simulink model "LoFT_Example3"  (R2024b)
settings: Solver=ode4  StartTime=0.0  StopTime=300  FixedStep=simu.dt  RelTol=1e-3
undefined symbols (not defined in the file): body, circtime, Communication, D1, Delta, irkb, line, LoFT, p0, Pn, s, simu, trip_time, Turbwind, waves, wind
libraries: simulink x350, spsThreePhaseVIMeasurementLib x41, spsThreePhasePISectionLineLib x34, spsThreePhaseParallelRLCLoadLib x21, spsThreePhaseTransformerTwoWindingsLib x14, spsLoadFlowBusLib x10, spsThreePhaseDynamicLoadLib x9, spsSynchronousMachinepuStandardLib x7, spsExcitationSystemLib x7, spsSteamTurbineandGovernorLib x7, spsGenericPowerSystemStabilizerLib x7, spsMultiBandPowerSystemStabilizerLib x7
(part 46 of 49)

== system LoFT_Example3/FOWT System/Subsystem13/FOWT2/Aerodynamics and Local Control Systems/Local Control Systems/Subsystem1/Gain Scheduling ==
  In1 : Inport
  In3 : Inport  Port=2
  In2 : Inport  Port=3
  1-D Lookup Table1 : Lookup_n-D  NumberOfTableDimensions=1  BreakpointsForDimension1=Controller.R.PC_GS_angles  Table=Controller.R.PC_GS_KI  InternalRulePriority=Speed  RndMeth=Simplest
  1-D Lookup Table2 : Lookup_n-D  NumberOfTableDimensions=1  BreakpointsForDimension1=Controller.R.PC_GS_angles  Table=Controller.R.PC_GS_KP  InternalRulePriority=Speed  RndMeth=Simplest
  Add : Sum
  Add1 : Sum
  Constant1 : Constant  Value=90*pi/180
  Delay : Delay  DelayLength=1  InitialCondition=0
  Gain : Gain  Gain=simu.dt
  Product : Product
  Product1 : Product
  Saturation Dynamic : simulink/Discontinuities/Saturation Dynamic  OutMin=[]  OutMax=[]  OutDataTypeStr=Inherit: Same as second input  OutDataType=fixdt(1, 16)  OutScaling=2^-10  DoSatur=off
  Saturation1 : Saturate  UpperLimit=Controller.R.PC_GS_KI(end)  LowerLimit=Controller.R.PC_GS_KI(1)
  Saturation3 : Saturate  UpperLimit=Controller.R.PC_GS_KP(end)  LowerLimit=Controller.R.PC_GS_KP(1)
  Out1 : Outport
  wires:
  Product/1 -> Add1/1
  Add1/1 -> Out1/1
  Delay/1 -> Add/2
  Saturation Dynamic/1 -> Delay/1, Add1/2
  Constant1/1 -> Saturation Dynamic/1
  In3/1 -> Saturation Dynamic/3
  Add/1 -> Saturation Dynamic/2
  Gain/1 -> Add/1
  Product1/1 -> Gain/1
  Saturation1/1 -> Product1/2
  Saturation3/1 -> Product/2
  In1/1 -> Product1/1, Product/1
  In2/1 -> 1-D Lookup Table2/1, 1-D Lookup Table1/1
  1-D Lookup Table2/1 -> Saturation3/1
  1-D Lookup Table1/1 -> Saturation1/1

== system LoFT_Example3/FOWT System/Subsystem13/FOWT3/Aerodynamics and Local Control Systems/Local Control Systems/Subsystem1/Gain Scheduling ==
  In1 : Inport
  In3 : Inport  Port=2
  In2 : Inport  Port=3
  1-D Lookup Table1 : Lookup_n-D  NumberOfTableDimensions=1  BreakpointsForDimension1=Controller.R.PC_GS_angles  Table=Controller.R.PC_GS_KI  InternalRulePriority=Speed  RndMeth=Simplest
  1-D Lookup Table2 : Lookup_n-D  NumberOfTableDimensions=1  BreakpointsForDimension1=Controller.R.PC_GS_angles  Table=Controller.R.PC_GS_KP  InternalRulePriority=Speed  RndMeth=Simplest
  Add : Sum
  Add1 : Sum
  Constant1 : Constant  Value=90*pi/180
  Delay : Delay  DelayLength=1  InitialCondition=0
  Gain : Gain  Gain=simu.dt
  Product : Product
  Product1 : Product
  Saturation Dynamic : simulink/Discontinuities/Saturation Dynamic  OutMin=[]  OutMax=[]  OutDataTypeStr=Inherit: Same as second input  OutDataType=fixdt(1, 16)  OutScaling=2^-10  DoSatur=off
  Saturation1 : Saturate  UpperLimit=Controller.R.PC_GS_KI(end)  LowerLimit=Controller.R.PC_GS_KI(1)
  Saturation3 : Saturate  UpperLimit=Controller.R.PC_GS_KP(end)  LowerLimit=Controller.R.PC_GS_KP(1)
  Out1 : Outport
  wires:
  1-D Lookup Table1/1 -> Saturation1/1
  1-D Lookup Table2/1 -> Saturation3/1
  In2/1 -> 1-D Lookup Table1/1, 1-D Lookup Table2/1
  In1/1 -> Product/1, Product1/1
  Saturation3/1 -> Product/2
  Saturation1/1 -> Product1/2
  Product1/1 -> Gain/1
  Gain/1 -> Add/1
  Add/1 -> Saturation Dynamic/2
  In3/1 -> Saturation Dynamic/3
  Constant1/1 -> Saturation Dynamic/1
  Saturation Dynamic/1 -> Add1/2, Delay/1
  Delay/1 -> Add/2
  Add1/1 -> Out1/1
  Product/1 -> Add1/1

== system LoFT_Example3/FOWT System/Subsystem13/FOWT4/Aerodynamics and Local Control Systems/Local Control Systems/Subsystem1/Gain Scheduling ==
  In1 : Inport
  In3 : Inport  Port=2
  In2 : Inport  Port=3
  1-D Lookup Table1 : Lookup_n-D  NumberOfTableDimensions=1  BreakpointsForDimension1=Controller.R.PC_GS_angles  Table=Controller.R.PC_GS_KI  InternalRulePriority=Speed  RndMeth=Simplest
  1-D Lookup Table2 : Lookup_n-D  NumberOfTableDimensions=1  BreakpointsForDimension1=Controller.R.PC_GS_angles  Table=Controller.R.PC_GS_KP  InternalRulePriority=Speed  RndMeth=Simplest
  Add : Sum
  Add1 : Sum
  Constant1 : Constant  Value=90*pi/180
  Delay : Delay  DelayLength=1  InitialCondition=0
  Gain : Gain  Gain=simu.dt
  Product : Product
  Product1 : Product
  Saturation Dynamic : simulink/Discontinuities/Saturation Dynamic  OutMin=[]  OutMax=[]  OutDataTypeStr=Inherit: Same as second input  OutDataType=fixdt(1, 16)  OutScaling=2^-10  DoSatur=off
  Saturation1 : Saturate  UpperLimit=Controller.R.PC_GS_KI(end)  LowerLimit=Controller.R.PC_GS_KI(1)
  Saturation3 : Saturate  UpperLimit=Controller.R.PC_GS_KP(end)  LowerLimit=Controller.R.PC_GS_KP(1)
  Out1 : Outport
  wires:
  Product/1 -> Add1/1
  Add1/1 -> Out1/1
  Delay/1 -> Add/2
  Saturation Dynamic/1 -> Delay/1, Add1/2
  Constant1/1 -> Saturation Dynamic/1
  In3/1 -> Saturation Dynamic/3
  Add/1 -> Saturation Dynamic/2
  Gain/1 -> Add/1
  Product1/1 -> Gain/1
  Saturation1/1 -> Product1/2
  Saturation3/1 -> Product/2
  In1/1 -> Product1/1, Product/1
  In2/1 -> 1-D Lookup Table2/1, 1-D Lookup Table1/1
  1-D Lookup Table2/1 -> Saturation3/1
  1-D Lookup Table1/1 -> Saturation1/1

== system LoFT_Example3/FOWT System/Subsystem13/FOWT5/Aerodynamics and Local Control Systems/Local Control Systems/Subsystem1/Gain Scheduling ==
  In1 : Inport
  In3 : Inport  Port=2
  In2 : Inport  Port=3
  1-D Lookup Table1 : Lookup_n-D  NumberOfTableDimensions=1  BreakpointsForDimension1=Controller.R.PC_GS_angles  Table=Controller.R.PC_GS_KI  InternalRulePriority=Speed  RndMeth=Simplest
  1-D Lookup Table2 : Lookup_n-D  NumberOfTableDimensions=1  BreakpointsForDimension1=Controller.R.PC_GS_angles  Table=Controller.R.PC_GS_KP  InternalRulePriority=Speed  RndMeth=Simplest
  Add : Sum
  Add1 : Sum
  Constant1 : Constant  Value=90*pi/180
  Delay : Delay  DelayLength=1  InitialCondition=0
  Gain : Gain  Gain=simu.dt
  Product : Product
  Product1 : Product
  Saturation Dynamic : simulink/Discontinuities/Saturation Dynamic  OutMin=[]  OutMax=[]  OutDataTypeStr=Inherit: Same as second input  OutDataType=fixdt(1, 16)  OutScaling=2^-10  DoSatur=off
  Saturation1 : Saturate  UpperLimit=Controller.R.PC_GS_KI(end)  LowerLimit=Controller.R.PC_GS_KI(1)
  Saturation3 : Saturate  UpperLimit=Controller.R.PC_GS_KP(end)  LowerLimit=Controller.R.PC_GS_KP(1)
  Out1 : Outport
  wires:
  1-D Lookup Table1/1 -> Saturation1/1
  1-D Lookup Table2/1 -> Saturation3/1
  In2/1 -> 1-D Lookup Table1/1, 1-D Lookup Table2/1
  In1/1 -> Product/1, Product1/1
  Saturation3/1 -> Product/2
  Saturation1/1 -> Product1/2
  Product1/1 -> Gain/1
  Gain/1 -> Add/1
  Add/1 -> Saturation Dynamic/2
  In3/1 -> Saturation Dynamic/3
  Constant1/1 -> Saturation Dynamic/1
  Saturation Dynamic/1 -> Add1/2, Delay/1
  Delay/1 -> Add/2
  Add1/1 -> Out1/1
  Product/1 -> Add1/1

== system LoFT_Example3/FOWT System/Subsystem13/FOWT6/Aerodynamics and Local Control Systems/Local Control Systems/Subsystem1/Gain Scheduling ==
  In1 : Inport
  In3 : Inport  Port=2
  In2 : Inport  Port=3
  1-D Lookup Table1 : Lookup_n-D  NumberOfTableDimensions=1  BreakpointsForDimension1=Controller.R.PC_GS_angles  Table=Controller.R.PC_GS_KI  InternalRulePriority=Speed  RndMeth=Simplest
  1-D Lookup Table2 : Lookup_n-D  NumberOfTableDimensions=1  BreakpointsForDimension1=Controller.R.PC_GS_angles  Table=Controller.R.PC_GS_KP  InternalRulePriority=Speed  RndMeth=Simplest
  Add : Sum
  Add1 : Sum
  Constant1 : Constant  Value=90*pi/180
  Delay : Delay  DelayLength=1  InitialCondition=0
  Gain : Gain  Gain=simu.dt
  Product : Product
  Product1 : Product
  Saturation Dynamic : simulink/Discontinuities/Saturation Dynamic  OutMin=[]  OutMax=[]  OutDataTypeStr=Inherit: Same as second input  OutDataType=fixdt(1, 16)  OutScaling=2^-10  DoSatur=off
  Saturation1 : Saturate  UpperLimit=Controller.R.PC_GS_KI(end)  LowerLimit=Controller.R.PC_GS_KI(1)
  Saturation3 : Saturate  UpperLimit=Controller.R.PC_GS_KP(end)  LowerLimit=Controller.R.PC_GS_KP(1)
  Out1 : Outport
  wires:
  Product/1 -> Add1/1
  Add1/1 -> Out1/1
  Delay/1 -> Add/2
  Saturation Dynamic/1 -> Delay/1, Add1/2
  Constant1/1 -> Saturation Dynamic/1
  In3/1 -> Saturation Dynamic/3
  Add/1 -> Saturation Dynamic/2
  Gain/1 -> Add/1
  Product1/1 -> Gain/1
  Saturation1/1 -> Product1/2
  Saturation3/1 -> Product/2
  In1/1 -> Product1/1, Product/1
  In2/1 -> 1-D Lookup Table2/1, 1-D Lookup Table1/1
  1-D Lookup Table2/1 -> Saturation3/1
  1-D Lookup Table1/1 -> Saturation1/1

== system LoFT_Example3/FOWT System/Subsystem13/FOWT7/Aerodynamics and Local Control Systems/Local Control Systems/Subsystem1/Gain Scheduling ==
  In1 : Inport
  In3 : Inport  Port=2
  In2 : Inport  Port=3
  1-D Lookup Table1 : Lookup_n-D  NumberOfTableDimensions=1  BreakpointsForDimension1=Controller.R.PC_GS_angles  Table=Controller.R.PC_GS_KI  InternalRulePriority=Speed  RndMeth=Simplest
  1-D Lookup Table2 : Lookup_n-D  NumberOfTableDimensions=1  BreakpointsForDimension1=Controller.R.PC_GS_angles  Table=Controller.R.PC_GS_KP  InternalRulePriority=Speed  RndMeth=Simplest
  Add : Sum
  Add1 : Sum
  Constant1 : Constant  Value=90*pi/180
  Delay : Delay  DelayLength=1  InitialCondition=0
  Gain : Gain  Gain=simu.dt
  Product : Product
  Product1 : Product
  Saturation Dynamic : simulink/Discontinuities/Saturation Dynamic  OutMin=[]  OutMax=[]  OutDataTypeStr=Inherit: Same as second input  OutDataType=fixdt(1, 16)  OutScaling=2^-10  DoSatur=off
  Saturation1 : Saturate  UpperLimit=Controller.R.PC_GS_KI(end)  LowerLimit=Controller.R.PC_GS_KI(1)
  Saturation3 : Saturate  UpperLimit=Controller.R.PC_GS_KP(end)  LowerLimit=Controller.R.PC_GS_KP(1)
  Out1 : Outport
  wires:
  1-D Lookup Table1/1 -> Saturation1/1
  1-D Lookup Table2/1 -> Saturation3/1
  In2/1 -> 1-D Lookup Table1/1, 1-D Lookup Table2/1
  In1/1 -> Product/1, Product1/1
  Saturation3/1 -> Product/2
  Saturation1/1 -> Product1/2
  Product1/1 -> Gain/1
  Gain/1 -> Add/1
  Add/1 -> Saturation Dynamic/2
  In3/1 -> Saturation Dynamic/3
  Constant1/1 -> Saturation Dynamic/1
  Saturation Dynamic/1 -> Add1/2, Delay/1
  Delay/1 -> Add/2
  Add1/1 -> Out1/1
  Product/1 -> Add1/1

== system LoFT_Example3/FOWT System/Subsystem13/FOWT8/Aerodynamics and Local Control Systems/Local Control Systems/Subsystem1/Gain Scheduling ==
  In1 : Inport
  In3 : Inport  Port=2
  In2 : Inport  Port=3
  1-D Lookup Table1 : Lookup_n-D  NumberOfTableDimensions=1  BreakpointsForDimension1=Controller.R.PC_GS_angles  Table=Controller.R.PC_GS_KI  InternalRulePriority=Speed  RndMeth=Simplest
  1-D Lookup Table2 : Lookup_n-D  NumberOfTableDimensions=1  BreakpointsForDimension1=Controller.R.PC_GS_angles  Table=Controller.R.PC_GS_KP  InternalRulePriority=Speed  RndMeth=Simplest
  Add : Sum
  Add1 : Sum
  Constant1 : Constant  Value=90*pi/180
  Delay : Delay  DelayLength=1  InitialCondition=0
  Gain : Gain  Gain=simu.dt
  Product : Product
  Product1 : Product
  Saturation Dynamic : simulink/Discontinuities/Saturation Dynamic  OutMin=[]  OutMax=[]  OutDataTypeStr=Inherit: Same as second input  OutDataType=fixdt(1, 16)  OutScaling=2^-10  DoSatur=off
  Saturation1 : Saturate  UpperLimit=Controller.R.PC_GS_KI(end)  LowerLimit=Controller.R.PC_GS_KI(1)
  Saturation3 : Saturate  UpperLimit=Controller.R.PC_GS_KP(end)  LowerLimit=Controller.R.PC_GS_KP(1)
  Out1 : Outport
  wires:
  Product/1 -> Add1/1
  Add1/1 -> Out1/1
  Delay/1 -> Add/2
  Saturation Dynamic/1 -> Delay/1, Add1/2
  Constant1/1 -> Saturation Dynamic/1
  In3/1 -> Saturation Dynamic/3
  Add/1 -> Saturation Dynamic/2
  Gain/1 -> Add/1
  Product1/1 -> Gain/1
  Saturation1/1 -> Product1/2
  Saturation3/1 -> Product/2
  In1/1 -> Product1/1, Product/1
  In2/1 -> 1-D Lookup Table2/1, 1-D Lookup Table1/1
  1-D Lookup Table2/1 -> Saturation3/1
  1-D Lookup Table1/1 -> Saturation1/1

== system LoFT_Example3/FOWT System/Subsystem13/FOWT9/Aerodynamics and Local Control Systems/Local Control Systems/Subsystem1/Gain Scheduling ==
  In1 : Inport
  In3 : Inport  Port=2
  In2 : Inport  Port=3
  1-D Lookup Table1 : Lookup_n-D  NumberOfTableDimensions=1  BreakpointsForDimension1=Controller.R.PC_GS_angles  Table=Controller.R.PC_GS_KI  InternalRulePriority=Speed  RndMeth=Simplest
  1-D Lookup Table2 : Lookup_n-D  NumberOfTableDimensions=1  BreakpointsForDimension1=Controller.R.PC_GS_angles  Table=Controller.R.PC_GS_KP  InternalRulePriority=Speed  RndMeth=Simplest
  Add : Sum
  Add1 : Sum
  Constant1 : Constant  Value=90*pi/180
  Delay : Delay  DelayLength=1  InitialCondition=0
  Gain : Gain  Gain=simu.dt
  Product : Product
  Product1 : Product
  Saturation Dynamic : simulink/Discontinuities/Saturation Dynamic  OutMin=[]  OutMax=[]  OutDataTypeStr=Inherit: Same as second input  OutDataType=fixdt(1, 16)  OutScaling=2^-10  DoSatur=off
  Saturation1 : Saturate  UpperLimit=Controller.R.PC_GS_KI(end)  LowerLimit=Controller.R.PC_GS_KI(1)
  Saturation3 : Saturate  UpperLimit=Controller.R.PC_GS_KP(end)  LowerLimit=Controller.R.PC_GS_KP(1)
  Out1 : Outport
  wires:
  1-D Lookup Table1/1 -> Saturation1/1
  1-D Lookup Table2/1 -> Saturation3/1
  In2/1 -> 1-D Lookup Table1/1, 1-D Lookup Table2/1
  In1/1 -> Product/1, Product1/1
  Saturation3/1 -> Product/2
  Saturation1/1 -> Product1/2
  Product1/1 -> Gain/1
  Gain/1 -> Add/1
  Add/1 -> Saturation Dynamic/2
  In3/1 -> Saturation Dynamic/3
  Constant1/1 -> Saturation Dynamic/1
  Saturation Dynamic/1 -> Add1/2, Delay/1
  Delay/1 -> Add/2
  Add1/1 -> Out1/1
  Product/1 -> Add1/1

== system LoFT_Example3/FOWT System/Subsystem2/FOWT1/Aerodynamics and Local Control Systems/Local Control Systems/Subsystem1/Gain Scheduling ==
  In1 : Inport
  In3 : Inport  Port=2
  In2 : Inport  Port=3
  1-D Lookup Table1 : Lookup_n-D  NumberOfTableDimensions=1  BreakpointsForDimension1=Controller.R.PC_GS_angles  Table=Controller.R.PC_GS_KI  InternalRulePriority=Speed  RndMeth=Simplest
  1-D Lookup Table2 : Lookup_n-D  NumberOfTableDimensions=1  BreakpointsForDimension1=Controller.R.PC_GS_angles  Table=Controller.R.PC_GS_KP  InternalRulePriority=Speed  RndMeth=Simplest
  Add : Sum
  Add1 : Sum
  Constant1 : Constant  Value=90*pi/180
  Delay : Delay  DelayLength=1  InitialCondition=0
  Gain : Gain  Gain=simu.dt
  Product : Product
  Product1 : Product
  Saturation Dynamic : simulink/Discontinuities/Saturation Dynamic  OutMin=[]  OutMax=[]  OutDataTypeStr=Inherit: Same as second input  OutDataType=fixdt(1, 16)  OutScaling=2^-10  DoSatur=off
  Saturation1 : Saturate  UpperLimit=Controller.R.PC_GS_KI(end)  LowerLimit=Controller.R.PC_GS_KI(1)
  Saturation3 : Saturate  UpperLimit=Controller.R.PC_GS_KP(end)  LowerLimit=Controller.R.PC_GS_KP(1)
  Out1 : Outport
  wires:
  1-D Lookup Table1/1 -> Saturation1/1
  1-D Lookup Table2/1 -> Saturation3/1
  In2/1 -> 1-D Lookup Table1/1, 1-D Lookup Table2/1
  In1/1 -> Product/1, Product1/1
  Saturation3/1 -> Product/2
  Saturation1/1 -> Product1/2
  Product1/1 -> Gain/1
  Gain/1 -> Add/1
  Add/1 -> Saturation Dynamic/2
  In3/1 -> Saturation Dynamic/3
  Constant1/1 -> Saturation Dynamic/1
  Saturation Dynamic/1 -> Add1/2, Delay/1
  Delay/1 -> Add/2
  Add1/1 -> Out1/1
  Product/1 -> Add1/1

== system LoFT_Example3/FOWT System/Subsystem2/FOWT10/Aerodynamics and Local Control Systems/Local Control Systems/Subsystem1/Gain Scheduling ==
  In1 : Inport
  In3 : Inport  Port=2
  In2 : Inport  Port=3
  1-D Lookup Table1 : Lookup_n-D  NumberOfTableDimensions=1  BreakpointsForDimension1=Controller.R.PC_GS_angles  Table=Controller.R.PC_GS_KI  InternalRulePriority=Speed  RndMeth=Simplest
  1-D Lookup Table2 : Lookup_n-D  NumberOfTableDimensions=1  BreakpointsForDimension1=Controller.R.PC_GS_angles  Table=Controller.R.PC_GS_KP  InternalRulePriority=Speed  RndMeth=Simplest
  Add : Sum
  Add1 : Sum
  Constant1 : Constant  Value=90*pi/180
  Delay : Delay  DelayLength=1  InitialCondition=0
  Gain : Gain  Gain=simu.dt
  Product : Product
  Product1 : Product
  Saturation Dynamic : simulink/Discontinuities/Saturation Dynamic  OutMin=[]  OutMax=[]  OutDataTypeStr=Inherit: Same as second input  OutDataType=fixdt(1, 16)  OutScaling=2^-10  DoSatur=off
  Saturation1 : Saturate  UpperLimit=Controller.R.PC_GS_KI(end)  LowerLimit=Controller.R.PC_GS_KI(1)
  Saturation3 : Saturate  UpperLimit=Controller.R.PC_GS_KP(end)  LowerLimit=Controller.R.PC_GS_KP(1)
  Out1 : Outport
  wires:
  Product/1 -> Add1/1
  Add1/1 -> Out1/1
  Delay/1 -> Add/2
  Saturation Dynamic/1 -> Delay/1, Add1/2
  Constant1/1 -> Saturation Dynamic/1
  In3/1 -> Saturation Dynamic/3
  Add/1 -> Saturation Dynamic/2
  Gain/1 -> Add/1
  Product1/1 -> Gain/1
  Saturation1/1 -> Product1/2
  Saturation3/1 -> Product/2
  In1/1 -> Product1/1, Product/1
  In2/1 -> 1-D Lookup Table2/1, 1-D Lookup Table1/1
  1-D Lookup Table2/1 -> Saturation3/1
  1-D Lookup Table1/1 -> Saturation1/1

== system LoFT_Example3/FOWT System/Subsystem2/FOWT2/Aerodynamics and Local Control Systems/Local Control Systems/Subsystem1/Gain Scheduling ==
  In1 : Inport
  In3 : Inport  Port=2
  In2 : Inport  Port=3
  1-D Lookup Table1 : Lookup_n-D  NumberOfTableDimensions=1  BreakpointsForDimension1=Controller.R.PC_GS_angles  Table=Controller.R.PC_GS_KI  InternalRulePriority=Speed  RndMeth=Simplest
  1-D Lookup Table2 : Lookup_n-D  NumberOfTableDimensions=1  BreakpointsForDimension1=Controller.R.PC_GS_angles  Table=Controller.R.PC_GS_KP  InternalRulePriority=Speed  RndMeth=Simplest
  Add : Sum
  Add1 : Sum
  Constant1 : Constant  Value=90*pi/180
  Delay : Delay  DelayLength=1  InitialCondition=0
  Gain : Gain  Gain=simu.dt
  Product : Product
  Product1 : Product
  Saturation Dynamic : simulink/Discontinuities/Saturation Dynamic  OutMin=[]  OutMax=[]  OutDataTypeStr=Inherit: Same as second input  OutDataType=fixdt(1, 16)  OutScaling=2^-10  DoSatur=off
  Saturation1 : Saturate  UpperLimit=Controller.R.PC_GS_KI(end)  LowerLimit=Controller.R.PC_GS_KI(1)
  Saturation3 : Saturate  UpperLimit=Controller.R.PC_GS_KP(end)  LowerLimit=Controller.R.PC_GS_KP(1)
  Out1 : Outport
  wires:
  Product/1 -> Add1/1
  Add1/1 -> Out1/1
  Delay/1 -> Add/2
  Saturation Dynamic/1 -> Delay/1, Add1/2
  Constant1/1 -> Saturation Dynamic/1
  In3/1 -> Saturation Dynamic/3
  Add/1 -> Saturation Dynamic/2
  Gain/1 -> Add/1
  Product1/1 -> Gain/1
  Saturation1/1 -> Product1/2
  Saturation3/1 -> Product/2
  In1/1 -> Product1/1, Product/1
  In2/1 -> 1-D Lookup Table2/1, 1-D Lookup Table1/1
  1-D Lookup Table2/1 -> Saturation3/1
  1-D Lookup Table1/1 -> Saturation1/1

== system LoFT_Example3/FOWT System/Subsystem2/FOWT3/Aerodynamics and Local Control Systems/Local Control Systems/Subsystem1/Gain Scheduling ==
  In1 : Inport
  In3 : Inport  Port=2
  In2 : Inport  Port=3
  1-D Lookup Table1 : Lookup_n-D  NumberOfTableDimensions=1  BreakpointsForDimension1=Controller.R.PC_GS_angles  Table=Controller.R.PC_GS_KI  InternalRulePriority=Speed  RndMeth=Simplest
  1-D Lookup Table2 : Lookup_n-D  NumberOfTableDimensions=1  BreakpointsForDimension1=Controller.R.PC_GS_angles  Table=Controller.R.PC_GS_KP  InternalRulePriority=Speed  RndMeth=Simplest
  Add : Sum
  Add1 : Sum
  Constant1 : Constant  Value=90*pi/180
  Delay : Delay  DelayLength=1  InitialCondition=0
  Gain : Gain  Gain=simu.dt
  Product : Product
  Product1 : Product
  Saturation Dynamic : simulink/Discontinuities/Saturation Dynamic  OutMin=[]  OutMax=[]  OutDataTypeStr=Inherit: Same as second input  OutDataType=fixdt(1, 16)  OutScaling=2^-10  DoSatur=off
  Saturation1 : Saturate  UpperLimit=Controller.R.PC_GS_KI(end)  LowerLimit=Controller.R.PC_GS_KI(1)
  Saturation3 : Saturate  UpperLimit=Controller.R.PC_GS_KP(end)  LowerLimit=Controller.R.PC_GS_KP(1)
  Out1 : Outport
  wires:
  1-D Lookup Table1/1 -> Saturation1/1
  1-D Lookup Table2/1 -> Saturation3/1
  In2/1 -> 1-D Lookup Table1/1, 1-D Lookup Table2/1
  In1/1 -> Product/1, Product1/1
  Saturation3/1 -> Product/2
  Saturation1/1 -> Product1/2
  Product1/1 -> Gain/1
  Gain/1 -> Add/1
  Add/1 -> Saturation Dynamic/2
  In3/1 -> Saturation Dynamic/3
  Constant1/1 -> Saturation Dynamic/1
  Saturation Dynamic/1 -> Add1/2, Delay/1
  Delay/1 -> Add/2
  Add1/1 -> Out1/1
  Product/1 -> Add1/1

== system LoFT_Example3/FOWT System/Subsystem2/FOWT4/Aerodynamics and Local Control Systems/Local Control Systems/Subsystem1/Gain Scheduling ==
  In1 : Inport
  In3 : Inport  Port=2
  In2 : Inport  Port=3
  1-D Lookup Table1 : Lookup_n-D  NumberOfTableDimensions=1  BreakpointsForDimension1=Controller.R.PC_GS_angles  Table=Controller.R.PC_GS_KI  InternalRulePriority=Speed  RndMeth=Simplest
  1-D Lookup Table2 : Lookup_n-D  NumberOfTableDimensions=1  BreakpointsForDimension1=Controller.R.PC_GS_angles  Table=Controller.R.PC_GS_KP  InternalRulePriority=Speed  RndMeth=Simplest
  Add : Sum
  Add1 : Sum
  Constant1 : Constant  Value=90*pi/180
  Delay : Delay  DelayLength=1  InitialCondition=0
  Gain : Gain  Gain=simu.dt
  Product : Product
  Product1 : Product
  Saturation Dynamic : simulink/Discontinuities/Saturation Dynamic  OutMin=[]  OutMax=[]  OutDataTypeStr=Inherit: Same as second input  OutDataType=fixdt(1, 16)  OutScaling=2^-10  DoSatur=off
  Saturation1 : Saturate  UpperLimit=Controller.R.PC_GS_KI(end)  LowerLimit=Controller.R.PC_GS_KI(1)
  Saturation3 : Saturate  UpperLimit=Controller.R.PC_GS_KP(end)  LowerLimit=Controller.R.PC_GS_KP(1)
  Out1 : Outport
  wires:
  Product/1 -> Add1/1
  Add1/1 -> Out1/1
  Delay/1 -> Add/2
  Saturation Dynamic/1 -> Delay/1, Add1/2
  Constant1/1 -> Saturation Dynamic/1
  In3/1 -> Saturation Dynamic/3
  Add/1 -> Saturation Dynamic/2
  Gain/1 -> Add/1
  Product1/1 -> Gain/1
  Saturation1/1 -> Product1/2
  Saturation3/1 -> Product/2
  In1/1 -> Product1/1, Product/1
  In2/1 -> 1-D Lookup Table2/1, 1-D Lookup Table1/1
  1-D Lookup Table2/1 -> Saturation3/1
  1-D Lookup Table1/1 -> Saturation1/1

== system LoFT_Example3/FOWT System/Subsystem2/FOWT5/Aerodynamics and Local Control Systems/Local Control Systems/Subsystem1/Gain Scheduling ==
  In1 : Inport
  In3 : Inport  Port=2
  In2 : Inport  Port=3
  1-D Lookup Table1 : Lookup_n-D  NumberOfTableDimensions=1  BreakpointsForDimension1=Controller.R.PC_GS_angles  Table=Controller.R.PC_GS_KI  InternalRulePriority=Speed  RndMeth=Simplest
  1-D Lookup Table2 : Lookup_n-D  NumberOfTableDimensions=1  BreakpointsForDimension1=Controller.R.PC_GS_angles  Table=Controller.R.PC_GS_KP  InternalRulePriority=Speed  RndMeth=Simplest
  Add : Sum
  Add1 : Sum
  Constant1 : Constant  Value=90*pi/180
  Delay : Delay  DelayLength=1  InitialCondition=0
  Gain : Gain  Gain=simu.dt
  Product : Product
  Product1 : Product
  Saturation Dynamic : simulink/Discontinuities/Saturation Dynamic  OutMin=[]  OutMax=[]  OutDataTypeStr=Inherit: Same as second input  OutDataType=fixdt(1, 16)  OutScaling=2^-10  DoSatur=off
  Saturation1 : Saturate  UpperLimit=Controller.R.PC_GS_KI(end)  LowerLimit=Controller.R.PC_GS_KI(1)
  Saturation3 : Saturate  UpperLimit=Controller.R.PC_GS_KP(end)  LowerLimit=Controller.R.PC_GS_KP(1)
  Out1 : Outport
  wires:
  1-D Lookup Table1/1 -> Saturation1/1
  1-D Lookup Table2/1 -> Saturation3/1
  In2/1 -> 1-D Lookup Table1/1, 1-D Lookup Table2/1
  In1/1 -> Product/1, Product1/1
  Saturation3/1 -> Product/2
  Saturation1/1 -> Product1/2
  Product1/1 -> Gain/1
  Gain/1 -> Add/1
  Add/1 -> Saturation Dynamic/2
  In3/1 -> Saturation Dynamic/3
  Constant1/1 -> Saturation Dynamic/1
  Saturation Dynamic/1 -> Add1/2, Delay/1
  Delay/1 -> Add/2
  Add1/1 -> Out1/1
  Product/1 -> Add1/1

== system LoFT_Example3/FOWT System/Subsystem2/FOWT6/Aerodynamics and Local Control Systems/Local Control Systems/Subsystem1/Gain Scheduling ==
  In1 : Inport
  In3 : Inport  Port=2
  In2 : Inport  Port=3
  1-D Lookup Table1 : Lookup_n-D  NumberOfTableDimensions=1  BreakpointsForDimension1=Controller.R.PC_GS_angles  Table=Controller.R.PC_GS_KI  InternalRulePriority=Speed  RndMeth=Simplest
  1-D Lookup Table2 : Lookup_n-D  NumberOfTableDimensions=1  BreakpointsForDimension1=Controller.R.PC_GS_angles  Table=Controller.R.PC_GS_KP  InternalRulePriority=Speed  RndMeth=Simplest
  Add : Sum
  Add1 : Sum
  Constant1 : Constant  Value=90*pi/180
  Delay : Delay  DelayLength=1  InitialCondition=0
  Gain : Gain  Gain=simu.dt
  Product : Product
  Product1 : Product
  Saturation Dynamic : simulink/Discontinuities/Saturation Dynamic  OutMin=[]  OutMax=[]  OutDataTypeStr=Inherit: Same as second input  OutDataType=fixdt(1, 16)  OutScaling=2^-10  DoSatur=off
  Saturation1 : Saturate  UpperLimit=Controller.R.PC_GS_KI(end)  LowerLimit=Controller.R.PC_GS_KI(1)
  Saturation3 : Saturate  UpperLimit=Controller.R.PC_GS_KP(end)  LowerLimit=Controller.R.PC_GS_KP(1)
  Out1 : Outport
  wires:
  Product/1 -> Add1/1
  Add1/1 -> Out1/1
  Delay/1 -> Add/2
  Saturation Dynamic/1 -> Delay/1, Add1/2
  Constant1/1 -> Saturation Dynamic/1
  In3/1 -> Saturation Dynamic/3
  Add/1 -> Saturation Dynamic/2
  Gain/1 -> Add/1
  Product1/1 -> Gain/1
  Saturation1/1 -> Product1/2
  Saturation3/1 -> Product/2
  In1/1 -> Product1/1, Product/1
  In2/1 -> 1-D Lookup Table2/1, 1-D Lookup Table1/1
  1-D Lookup Table2/1 -> Saturation3/1
  1-D Lookup Table1/1 -> Saturation1/1

== system LoFT_Example3/FOWT System/Subsystem2/FOWT7/Aerodynamics and Local Control Systems/Local Control Systems/Subsystem1/Gain Scheduling ==
  In1 : Inport
  In3 : Inport  Port=2
  In2 : Inport  Port=3
  1-D Lookup Table1 : Lookup_n-D  NumberOfTableDimensions=1  BreakpointsForDimension1=Controller.R.PC_GS_angles  Table=Controller.R.PC_GS_KI  InternalRulePriority=Speed  RndMeth=Simplest
  1-D Lookup Table2 : Lookup_n-D  NumberOfTableDimensions=1  BreakpointsForDimension1=Controller.R.PC_GS_angles  Table=Controller.R.PC_GS_KP  InternalRulePriority=Speed  RndMeth=Simplest
  Add : Sum
  Add1 : Sum
  Constant1 : Constant  Value=90*pi/180
  Delay : Delay  DelayLength=1  InitialCondition=0
  Gain : Gain  Gain=simu.dt
  Product : Product
  Product1 : Product
  Saturation Dynamic : simulink/Discontinuities/Saturation Dynamic  OutMin=[]  OutMax=[]  OutDataTypeStr=Inherit: Same as second input  OutDataType=fixdt(1, 16)  OutScaling=2^-10  DoSatur=off
  Saturation1 : Saturate  UpperLimit=Controller.R.PC_GS_KI(end)  LowerLimit=Controller.R.PC_GS_KI(1)
  Saturation3 : Saturate  UpperLimit=Controller.R.PC_GS_KP(end)  LowerLimit=Controller.R.PC_GS_KP(1)
  Out1 : Outport
  wires:
  1-D Lookup Table1/1 -> Saturation1/1
  1-D Lookup Table2/1 -> Saturation3/1
  In2/1 -> 1-D Lookup Table1/1, 1-D Lookup Table2/1
  In1/1 -> Product/1, Product1/1
  Saturation3/1 -> Product/2
  Saturation1/1 -> Product1/2
  Product1/1 -> Gain/1
  Gain/1 -> Add/1
  Add/1 -> Saturation Dynamic/2
  In3/1 -> Saturation Dynamic/3
  Constant1/1 -> Saturation Dynamic/1
  Saturation Dynamic/1 -> Add1/2, Delay/1
  Delay/1 -> Add/2
  Add1/1 -> Out1/1
  Product/1 -> Add1/1

== system LoFT_Example3/FOWT System/Subsystem2/FOWT8/Aerodynamics and Local Control Systems/Local Control Systems/Subsystem1/Gain Scheduling ==
  In1 : Inport
  In3 : Inport  Port=2
  In2 : Inport  Port=3
  1-D Lookup Table1 : Lookup_n-D  NumberOfTableDimensions=1  BreakpointsForDimension1=Controller.R.PC_GS_angles  Table=Controller.R.PC_GS_KI  InternalRulePriority=Speed  RndMeth=Simplest
  1-D Lookup Table2 : Lookup_n-D  NumberOfTableDimensions=1  BreakpointsForDimension1=Controller.R.PC_GS_angles  Table=Controller.R.PC_GS_KP  InternalRulePriority=Speed  RndMeth=Simplest
  Add : Sum
  Add1 : Sum
  Constant1 : Constant  Value=90*pi/180
  Delay : Delay  DelayLength=1  InitialCondition=0
  Gain : Gain  Gain=simu.dt
  Product : Product
  Product1 : Product
  Saturation Dynamic : simulink/Discontinuities/Saturation Dynamic  OutMin=[]  OutMax=[]  OutDataTypeStr=Inherit: Same as second input  OutDataType=fixdt(1, 16)  OutScaling=2^-10  DoSatur=off
  Saturation1 : Saturate  UpperLimit=Controller.R.PC_GS_KI(end)  LowerLimit=Controller.R.PC_GS_KI(1)
  Saturation3 : Saturate  UpperLimit=Controller.R.PC_GS_KP(end)  LowerLimit=Controller.R.PC_GS_KP(1)
  Out1 : Outport
  wires:
  Product/1 -> Add1/1
  Add1/1 -> Out1/1
  Delay/1 -> Add/2
  Saturation Dynamic/1 -> Delay/1, Add1/2
  Constant1/1 -> Saturation Dynamic/1
  In3/1 -> Saturation Dynamic/3
  Add/1 -> Saturation Dynamic/2
  Gain/1 -> Add/1
  Product1/1 -> Gain/1
  Saturation1/1 -> Product1/2
  Saturation3/1 -> Product/2
  In1/1 -> Product1/1, Product/1
  In2/1 -> 1-D Lookup Table2/1, 1-D Lookup Table1/1
  1-D Lookup Table2/1 -> Saturation3/1
  1-D Lookup Table1/1 -> Saturation1/1

== system LoFT_Example3/FOWT System/Subsystem2/FOWT9/Aerodynamics and Local Control Systems/Local Control Systems/Subsystem1/Gain Scheduling ==
  In1 : Inport
  In3 : Inport  Port=2
  In2 : Inport  Port=3
  1-D Lookup Table1 : Lookup_n-D  NumberOfTableDimensions=1  BreakpointsForDimension1=Controller.R.PC_GS_angles  Table=Controller.R.PC_GS_KI  InternalRulePriority=Speed  RndMeth=Simplest
  1-D Lookup Table2 : Lookup_n-D  NumberOfTableDimensions=1  BreakpointsForDimension1=Controller.R.PC_GS_angles  Table=Controller.R.PC_GS_KP  InternalRulePriority=Speed  RndMeth=Simplest
  Add : Sum
  Add1 : Sum
  Constant1 : Constant  Value=90*pi/180
  Delay : Delay  DelayLength=1  InitialCondition=0
  Gain : Gain  Gain=simu.dt
  Product : Product
  Product1 : Product
  Saturation Dynamic : simulink/Discontinuities/Saturation Dynamic  OutMin=[]  OutMax=[]  OutDataTypeStr=Inherit: Same as second input  OutDataType=fixdt(1, 16)  OutScaling=2^-10  DoSatur=off
  Saturation1 : Saturate  UpperLimit=Controller.R.PC_GS_KI(end)  LowerLimit=Controller.R.PC_GS_KI(1)
  Saturation3 : Saturate  UpperLimit=Controller.R.PC_GS_KP(end)  LowerLimit=Controller.R.PC_GS_KP(1)
  Out1 : Outport
  wires:
  1-D Lookup Table1/1 -> Saturation1/1
  1-D Lookup Table2/1 -> Saturation3/1
  In2/1 -> 1-D Lookup Table1/1, 1-D Lookup Table2/1
  In1/1 -> Product/1, Product1/1
  Saturation3/1 -> Product/2
  Saturation1/1 -> Product1/2
  Product1/1 -> Gain/1
  Gain/1 -> Add/1
  Add/1 -> Saturation Dynamic/2
  In3/1 -> Saturation Dynamic/3
  Constant1/1 -> Saturation Dynamic/1
  Saturation Dynamic/1 -> Add1/2, Delay/1
  Delay/1 -> Add/2
  Add1/1 -> Out1/1
  Product/1 -> Add1/1

== system LoFT_Example3/FOWT System/Subsystem3/FOWT1/Aerodynamics and Local Control Systems/Local Control Systems/Subsystem1/Gain Scheduling ==
  In1 : Inport
  In3 : Inport  Port=2
  In2 : Inport  Port=3
  1-D Lookup Table1 : Lookup_n-D  NumberOfTableDimensions=1  BreakpointsForDimension1=Controller.R.PC_GS_angles  Table=Controller.R.PC_GS_KI  InternalRulePriority=Speed  RndMeth=Simplest
  1-D Lookup Table2 : Lookup_n-D  NumberOfTableDimensions=1  BreakpointsForDimension1=Controller.R.PC_GS_angles  Table=Controller.R.PC_GS_KP  InternalRulePriority=Speed  RndMeth=Simplest
  Add : Sum
  Add1 : Sum
  Constant1 : Constant  Value=90*pi/180
  Delay : Delay  DelayLength=1  InitialCondition=0
  Gain : Gain  Gain=simu.dt
  Product : Product
  Product1 : Product
  Saturation Dynamic : simulink/Discontinuities/Saturation Dynamic  OutMin=[]  OutMax=[]  OutDataTypeStr=Inherit: Same as second input  OutDataType=fixdt(1, 16)  OutScaling=2^-10  DoSatur=off
  Saturation1 : Saturate  UpperLimit=Controller.R.PC_GS_KI(end)  LowerLimit=Controller.R.PC_GS_KI(1)
  Saturation3 : Saturate  UpperLimit=Controller.R.PC_GS_KP(end)  LowerLimit=Controller.R.PC_GS_KP(1)
  Out1 : Outport
  wires:
  Product/1 -> Add1/1
  Add1/1 -> Out1/1
  Delay/1 -> Add/2
  Saturation Dynamic/1 -> Delay/1, Add1/2
  Constant1/1 -> Saturation Dynamic/1
  In3/1 -> Saturation Dynamic/3
  Add/1 -> Saturation Dynamic/2
  Gain/1 -> Add/1
  Product1/1 -> Gain/1
  Saturation1/1 -> Product1/2
  Saturation3/1 -> Product/2
  In1/1 -> Product1/1, Product/1
  In2/1 -> 1-D Lookup Table2/1, 1-D Lookup Table1/1
  1-D Lookup Table2/1 -> Saturation3/1
  1-D Lookup Table1/1 -> Saturation1/1

== system LoFT_Example3/FOWT System/Subsystem3/FOWT10/Aerodynamics and Local Control Systems/Local Control Systems/Subsystem1/Gain Scheduling ==
  In1 : Inport
  In3 : Inport  Port=2
  In2 : Inport  Port=3
  1-D Lookup Table1 : Lookup_n-D  NumberOfTableDimensions=1  BreakpointsForDimension1=Controller.R.PC_GS_angles  Table=Controller.R.PC_GS_KI  InternalRulePriority=Speed  RndMeth=Simplest
  1-D Lookup Table2 : Lookup_n-D  NumberOfTableDimensions=1  BreakpointsForDimension1=Controller.R.PC_GS_angles  Table=Controller.R.PC_GS_KP  InternalRulePriority=Speed  RndMeth=Simplest
  Add : Sum
  Add1 : Sum
  Constant1 : Constant  Value=90*pi/180
  Delay : Delay  DelayLength=1  InitialCondition=0
  Gain : Gain  Gain=simu.dt
  Product : Product
  Product1 : Product
  Saturation Dynamic : simulink/Discontinuities/Saturation Dynamic  OutMin=[]  OutMax=[]  OutDataTypeStr=Inherit: Same as second input  OutDataType=fixdt(1, 16)  OutScaling=2^-10  DoSatur=off
  Saturation1 : Saturate  UpperLimit=Controller.R.PC_GS_KI(end)  LowerLimit=Controller.R.PC_GS_KI(1)
  Saturation3 : Saturate  UpperLimit=Controller.R.PC_GS_KP(end)  LowerLimit=Controller.R.PC_GS_KP(1)
  Out1 : Outport
  wires:
  1-D Lookup Table1/1 -> Saturation1/1
  1-D Lookup Table2/1 -> Saturation3/1
  In2/1 -> 1-D Lookup Table1/1, 1-D Lookup Table2/1
  In1/1 -> Product/1, Product1/1
  Saturation3/1 -> Product/2
  Saturation1/1 -> Product1/2
  Product1/1 -> Gain/1
  Gain/1 -> Add/1
  Add/1 -> Saturation Dynamic/2
  In3/1 -> Saturation Dynamic/3
  Constant1/1 -> Saturation Dynamic/1
  Saturation Dynamic/1 -> Add1/2, Delay/1
  Delay/1 -> Add/2
  Add1/1 -> Out1/1
  Product/1 -> Add1/1

== system LoFT_Example3/FOWT System/Subsystem3/FOWT2/Aerodynamics and Local Control Systems/Local Control Systems/Subsystem1/Gain Scheduling ==
  In1 : Inport
  In3 : Inport  Port=2
  In2 : Inport  Port=3
  1-D Lookup Table1 : Lookup_n-D  NumberOfTableDimensions=1  BreakpointsForDimension1=Controller.R.PC_GS_angles  Table=Controller.R.PC_GS_KI  InternalRulePriority=Speed  RndMeth=Simplest
  1-D Lookup Table2 : Lookup_n-D  NumberOfTableDimensions=1  BreakpointsForDimension1=Controller.R.PC_GS_angles  Table=Controller.R.PC_GS_KP  InternalRulePriority=Speed  RndMeth=Simplest
  Add : Sum
  Add1 : Sum
  Constant1 : Constant  Value=90*pi/180
  Delay : Delay  DelayLength=1  InitialCondition=0
  Gain : Gain  Gain=simu.dt
  Product : Product
  Product1 : Product
  Saturation Dynamic : simulink/Discontinuities/Saturation Dynamic  OutMin=[]  OutMax=[]  OutDataTypeStr=Inherit: Same as second input  OutDataType=fixdt(1, 16)  OutScaling=2^-10  DoSatur=off
  Saturation1 : Saturate  UpperLimit=Controller.R.PC_GS_KI(end)  LowerLimit=Controller.R.PC_GS_KI(1)
  Saturation3 : Saturate  UpperLimit=Controller.R.PC_GS_KP(end)  LowerLimit=Controller.R.PC_GS_KP(1)
  Out1 : Outport
  wires:
  1-D Lookup Table1/1 -> Saturation1/1
  1-D Lookup Table2/1 -> Saturation3/1
  In2/1 -> 1-D Lookup Table1/1, 1-D Lookup Table2/1
  In1/1 -> Product/1, Product1/1
  Saturation3/1 -> Product/2
  Saturation1/1 -> Product1/2
  Product1/1 -> Gain/1
  Gain/1 -> Add/1
  Add/1 -> Saturation Dynamic/2
  In3/1 -> Saturation Dynamic/3
  Constant1/1 -> Saturation Dynamic/1
  Saturation Dynamic/1 -> Add1/2, Delay/1
  Delay/1 -> Add/2
  Add1/1 -> Out1/1
  Product/1 -> Add1/1

== system LoFT_Example3/FOWT System/Subsystem3/FOWT3/Aerodynamics and Local Control Systems/Local Control Systems/Subsystem1/Gain Scheduling ==
  In1 : Inport
  In3 : Inport  Port=2
  In2 : Inport  Port=3
  1-D Lookup Table1 : Lookup_n-D  NumberOfTableDimensions=1  BreakpointsForDimension1=Controller.R.PC_GS_angles  Table=Controller.R.PC_GS_KI  InternalRulePriority=Speed  RndMeth=Simplest
  1-D Lookup Table2 : Lookup_n-D  NumberOfTableDimensions=1  BreakpointsForDimension1=Controller.R.PC_GS_angles  Table=Controller.R.PC_GS_KP  InternalRulePriority=Speed  RndMeth=Simplest
  Add : Sum
  Add1 : Sum
  Constant1 : Constant  Value=90*pi/180
  Delay : Delay  DelayLength=1  InitialCondition=0
  Gain : Gain  Gain=simu.dt
  Product : Product
  Product1 : Product
  Saturation Dynamic : simulink/Discontinuities/Saturation Dynamic  OutMin=[]  OutMax=[]  OutDataTypeStr=Inherit: Same as second input  OutDataType=fixdt(1, 16)  OutScaling=2^-10  DoSatur=off
  Saturation1 : Saturate  UpperLimit=Controller.R.PC_GS_KI(end)  LowerLimit=Controller.R.PC_GS_KI(1)
  Saturation3 : Saturate  UpperLimit=Controller.R.PC_GS_KP(end)  LowerLimit=Controller.R.PC_GS_KP(1)
  Out1 : Outport
  wires:
  Product/1 -> Add1/1
  Add1/1 -> Out1/1
  Delay/1 -> Add/2
  Saturation Dynamic/1 -> Delay/1, Add1/2
  Constant1/1 -> Saturation Dynamic/1
  In3/1 -> Saturation Dynamic/3
  Add/1 -> Saturation Dynamic/2
  Gain/1 -> Add/1
  Product1/1 -> Gain/1
  Saturation1/1 -> Product1/2
  Saturation3/1 -> Product/2
  In1/1 -> Product1/1, Product/1
  In2/1 -> 1-D Lookup Table2/1, 1-D Lookup Table1/1
  1-D Lookup Table2/1 -> Saturation3/1
  1-D Lookup Table1/1 -> Saturation1/1

== system LoFT_Example3/FOWT System/Subsystem3/FOWT4/Aerodynamics and Local Control Systems/Local Control Systems/Subsystem1/Gain Scheduling ==
  In1 : Inport
  In3 : Inport  Port=2
  In2 : Inport  Port=3
  1-D Lookup Table1 : Lookup_n-D  NumberOfTableDimensions=1  BreakpointsForDimension1=Controller.R.PC_GS_angles  Table=Controller.R.PC_GS_KI  InternalRulePriority=Speed  RndMeth=Simplest
  1-D Lookup Table2 : Lookup_n-D  NumberOfTableDimensions=1  BreakpointsForDimension1=Controller.R.PC_GS_angles  Table=Controller.R.PC_GS_KP  InternalRulePriority=Speed  RndMeth=Simplest
  Add : Sum
  Add1 : Sum
  Constant1 : Constant  Value=90*pi/180
  Delay : Delay  DelayLength=1  InitialCondition=0
  Gain : Gain  Gain=simu.dt
  Product : Product
  Product1 : Product
  Saturation Dynamic : simulink/Discontinuities/Saturation Dynamic  OutMin=[]  OutMax=[]  OutDataTypeStr=Inherit: Same as second input  OutDataType=fixdt(1, 16)  OutScaling=2^-10  DoSatur=off
  Saturation1 : Saturate  UpperLimit=Controller.R.PC_GS_KI(end)  LowerLimit=Controller.R.PC_GS_KI(1)
  Saturation3 : Saturate  UpperLimit=Controller.R.PC_GS_KP(end)  LowerLimit=Controller.R.PC_GS_KP(1)
  Out1 : Outport
  wires:
  1-D Lookup Table1/1 -> Saturation1/1
  1-D Lookup Table2/1 -> Saturation3/1
  In2/1 -> 1-D Lookup Table1/1, 1-D Lookup Table2/1
  In1/1 -> Product/1, Product1/1
  Saturation3/1 -> Product/2
  Saturation1/1 -> Product1/2
  Product1/1 -> Gain/1
  Gain/1 -> Add/1
  Add/1 -> Saturation Dynamic/2
  In3/1 -> Saturation Dynamic/3
  Constant1/1 -> Saturation Dynamic/1
  Saturation Dynamic/1 -> Add1/2, Delay/1
  Delay/1 -> Add/2
  Add1/1 -> Out1/1
  Product/1 -> Add1/1

== system LoFT_Example3/FOWT System/Subsystem3/FOWT5/Aerodynamics and Local Control Systems/Local Control Systems/Subsystem1/Gain Scheduling ==
  In1 : Inport
  In3 : Inport  Port=2
  In2 : Inport  Port=3
  1-D Lookup Table1 : Lookup_n-D  NumberOfTableDimensions=1  BreakpointsForDimension1=Controller.R.PC_GS_angles  Table=Controller.R.PC_GS_KI  InternalRulePriority=Speed  RndMeth=Simplest
  1-D Lookup Table2 : Lookup_n-D  NumberOfTableDimensions=1  BreakpointsForDimension1=Controller.R.PC_GS_angles  Table=Controller.R.PC_GS_KP  InternalRulePriority=Speed  RndMeth=Simplest
  Add : Sum
  Add1 : Sum
  Constant1 : Constant  Value=90*pi/180
  Delay : Delay  DelayLength=1  InitialCondition=0
  Gain : Gain  Gain=simu.dt
  Product : Product
  Product1 : Product
  Saturation Dynamic : simulink/Discontinuities/Saturation Dynamic  OutMin=[]  OutMax=[]  OutDataTypeStr=Inherit: Same as second input  OutDataType=fixdt(1, 16)  OutScaling=2^-10  DoSatur=off
  Saturation1 : Saturate  UpperLimit=Controller.R.PC_GS_KI(end)  LowerLimit=Controller.R.PC_GS_KI(1)
  Saturation3 : Saturate  UpperLimit=Controller.R.PC_GS_KP(end)  LowerLimit=Controller.R.PC_GS_KP(1)
  Out1 : Outport
  wires:
  Product/1 -> Add1/1
  Add1/1 -> Out1/1
  Delay/1 -> Add/2
  Saturation Dynamic/1 -> Delay/1, Add1/2
  Constant1/1 -> Saturation Dynamic/1
  In3/1 -> Saturation Dynamic/3
  Add/1 -> Saturation Dynamic/2
  Gain/1 -> Add/1
  Product1/1 -> Gain/1
  Saturation1/1 -> Product1/2
  Saturation3/1 -> Product/2
  In1/1 -> Product1/1, Product/1
  In2/1 -> 1-D Lookup Table2/1, 1-D Lookup Table1/1
  1-D Lookup Table2/1 -> Saturation3/1
  1-D Lookup Table1/1 -> Saturation1/1

== system LoFT_Example3/FOWT System/Subsystem3/FOWT6/Aerodynamics and Local Control Systems/Local Control Systems/Subsystem1/Gain Scheduling ==
  In1 : Inport
  In3 : Inport  Port=2
  In2 : Inport  Port=3
  1-D Lookup Table1 : Lookup_n-D  NumberOfTableDimensions=1  BreakpointsForDimension1=Controller.R.PC_GS_angles  Table=Controller.R.PC_GS_KI  InternalRulePriority=Speed  RndMeth=Simplest
  1-D Lookup Table2 : Lookup_n-D  NumberOfTableDimensions=1  BreakpointsForDimension1=Controller.R.PC_GS_angles  Table=Controller.R.PC_GS_KP  InternalRulePriority=Speed  RndMeth=Simplest
  Add : Sum
  Add1 : Sum
  Constant1 : Constant  Value=90*pi/180
  Delay : Delay  DelayLength=1  InitialCondition=0
  Gain : Gain  Gain=simu.dt
  Product : Product
  Product1 : Product
  Saturation Dynamic : simulink/Discontinuities/Saturation Dynamic  OutMin=[]  OutMax=[]  OutDataTypeStr=Inherit: Same as second input  OutDataType=fixdt(1, 16)  OutScaling=2^-10  DoSatur=off
  Saturation1 : Saturate  UpperLimit=Controller.R.PC_GS_KI(end)  LowerLimit=Controller.R.PC_GS_KI(1)
  Saturation3 : Saturate  UpperLimit=Controller.R.PC_GS_KP(end)  LowerLimit=Controller.R.PC_GS_KP(1)
  Out1 : Outport
  wires:
  1-D Lookup Table1/1 -> Saturation1/1
  1-D Lookup Table2/1 -> Saturation3/1
  In2/1 -> 1-D Lookup Table1/1, 1-D Lookup Table2/1
  In1/1 -> Product/1, Product1/1
  Saturation3/1 -> Product/2
  Saturation1/1 -> Product1/2
  Product1/1 -> Gain/1
  Gain/1 -> Add/1
  Add/1 -> Saturation Dynamic/2
  In3/1 -> Saturation Dynamic/3
  Constant1/1 -> Saturation Dynamic/1
  Saturation Dynamic/1 -> Add1/2, Delay/1
  Delay/1 -> Add/2
  Add1/1 -> Out1/1
  Product/1 -> Add1/1

== system LoFT_Example3/FOWT System/Subsystem3/FOWT7/Aerodynamics and Local Control Systems/Local Control Systems/Subsystem1/Gain Scheduling ==
  In1 : Inport
  In3 : Inport  Port=2
  In2 : Inport  Port=3
  1-D Lookup Table1 : Lookup_n-D  NumberOfTableDimensions=1  BreakpointsForDimension1=Controller.R.PC_GS_angles  Table=Controller.R.PC_GS_KI  InternalRulePriority=Speed  RndMeth=Simplest
  1-D Lookup Table2 : Lookup_n-D  NumberOfTableDimensions=1  BreakpointsForDimension1=Controller.R.PC_GS_angles  Table=Controller.R.PC_GS_KP  InternalRulePriority=Speed  RndMeth=Simplest
  Add : Sum
  Add1 : Sum
  Constant1 : Constant  Value=90*pi/180
  Delay : Delay  DelayLength=1  InitialCondition=0
  Gain : Gain  Gain=simu.dt
  Product : Product
  Product1 : Product
  Saturation Dynamic : simulink/Discontinuities/Saturation Dynamic  OutMin=[]  OutMax=[]  OutDataTypeStr=Inherit: Same as second input  OutDataType=fixdt(1, 16)  OutScaling=2^-10  DoSatur=off
  Saturation1 : Saturate  UpperLimit=Controller.R.PC_GS_KI(end)  LowerLimit=Controller.R.PC_GS_KI(1)
  Saturation3 : Saturate  UpperLimit=Controller.R.PC_GS_KP(end)  LowerLimit=Controller.R.PC_GS_KP(1)
  Out1 : Outport
  wires:
  Product/1 -> Add1/1
  Add1/1 -> Out1/1
  Delay/1 -> Add/2
  Saturation Dynamic/1 -> Delay/1, Add1/2
  Constant1/1 -> Saturation Dynamic/1
  In3/1 -> Saturation Dynamic/3
  Add/1 -> Saturation Dynamic/2
  Gain/1 -> Add/1
  Product1/1 -> Gain/1
  Saturation1/1 -> Product1/2
  Saturation3/1 -> Product/2
  In1/1 -> Product1/1, Product/1
  In2/1 -> 1-D Lookup Table2/1, 1-D Lookup Table1/1
  1-D Lookup Table2/1 -> Saturation3/1
  1-D Lookup Table1/1 -> Saturation1/1

== system LoFT_Example3/FOWT System/Subsystem3/FOWT8/Aerodynamics and Local Control Systems/Local Control Systems/Subsystem1/Gain Scheduling ==
  In1 : Inport
  In3 : Inport  Port=2
  In2 : Inport  Port=3
  1-D Lookup Table1 : Lookup_n-D  NumberOfTableDimensions=1  BreakpointsForDimension1=Controller.R.PC_GS_angles  Table=Controller.R.PC_GS_KI  InternalRulePriority=Speed  RndMeth=Simplest
  1-D Lookup Table2 : Lookup_n-D  NumberOfTableDimensions=1  BreakpointsForDimension1=Controller.R.PC_GS_angles  Table=Controller.R.PC_GS_KP  InternalRulePriority=Speed  RndMeth=Simplest
  Add : Sum
  Add1 : Sum
  Constant1 : Constant  Value=90*pi/180
  Delay : Delay  DelayLength=1  InitialCondition=0
  Gain : Gain  Gain=simu.dt
  Product : Product
  Product1 : Product
  Saturation Dynamic : simulink/Discontinuities/Saturation Dynamic  OutMin=[]  OutMax=[]  OutDataTypeStr=Inherit: Same as second input  OutDataType=fixdt(1, 16)  OutScaling=2^-10  DoSatur=off
  Saturation1 : Saturate  UpperLimit=Controller.R.PC_GS_KI(end)  LowerLimit=Controller.R.PC_GS_KI(1)
  Saturation3 : Saturate  UpperLimit=Controller.R.PC_GS_KP(end)  LowerLimit=Controller.R.PC_GS_KP(1)
  Out1 : Outport
  wires:
  1-D Lookup Table1/1 -> Saturation1/1
  1-D Lookup Table2/1 -> Saturation3/1
  In2/1 -> 1-D Lookup Table1/1, 1-D Lookup Table2/1
  In1/1 -> Product/1, Product1/1
  Saturation3/1 -> Product/2
  Saturation1/1 -> Product1/2
  Product1/1 -> Gain/1
  Gain/1 -> Add/1
  Add/1 -> Saturation Dynamic/2
  In3/1 -> Saturation Dynamic/3
  Constant1/1 -> Saturation Dynamic/1
  Saturation Dynamic/1 -> Add1/2, Delay/1
  Delay/1 -> Add/2
  Add1/1 -> Out1/1
  Product/1 -> Add1/1

== system LoFT_Example3/FOWT System/Subsystem3/FOWT9/Aerodynamics and Local Control Systems/Local Control Systems/Subsystem1/Gain Scheduling ==
  In1 : Inport
  In3 : Inport  Port=2
  In2 : Inport  Port=3
  1-D Lookup Table1 : Lookup_n-D  NumberOfTableDimensions=1  BreakpointsForDimension1=Controller.R.PC_GS_angles  Table=Controller.R.PC_GS_KI  InternalRulePriority=Speed  RndMeth=Simplest
  1-D Lookup Table2 : Lookup_n-D  NumberOfTableDimensions=1  BreakpointsForDimension1=Controller.R.PC_GS_angles  Table=Controller.R.PC_GS_KP  InternalRulePriority=Speed  RndMeth=Simplest
  Add : Sum
  Add1 : Sum
  Constant1 : Constant  Value=90*pi/180
  Delay : Delay  DelayLength=1  InitialCondition=0
  Gain : Gain  Gain=simu.dt
  Product : Product
  Product1 : Product
  Saturation Dynamic : simulink/Discontinuities/Saturation Dynamic  OutMin=[]  OutMax=[]  OutDataTypeStr=Inherit: Same as second input  OutDataType=fixdt(1, 16)  OutScaling=2^-10  DoSatur=off
  Saturation1 : Saturate  UpperLimit=Controller.R.PC_GS_KI(end)  LowerLimit=Controller.R.PC_GS_KI(1)
  Saturation3 : Saturate  UpperLimit=Controller.R.PC_GS_KP(end)  LowerLimit=Controller.R.PC_GS_KP(1)
  Out1 : Outport
  wires:
  Product/1 -> Add1/1
  Add1/1 -> Out1/1
  Delay/1 -> Add/2
  Saturation Dynamic/1 -> Delay/1, Add1/2
  Constant1/1 -> Saturation Dynamic/1
  In3/1 -> Saturation Dynamic/3
  Add/1 -> Saturation Dynamic/2
  Gain/1 -> Add/1
  Product1/1 -> Gain/1
  Saturation1/1 -> Product1/2
  Saturation3/1 -> Product/2
  In1/1 -> Product1/1, Product/1
  In2/1 -> 1-D Lookup Table2/1, 1-D Lookup Table1/1
  1-D Lookup Table2/1 -> Saturation3/1
  1-D Lookup Table1/1 -> Saturation1/1

== system LoFT_Example3/FOWT System/Subsystem5/FOWT1/Aerodynamics and Local Control Systems/Local Control Systems/Subsystem1/Gain Scheduling ==
  In1 : Inport
  In3 : Inport  Port=2
  In2 : Inport  Port=3
  1-D Lookup Table1 : Lookup_n-D  NumberOfTableDimensions=1  BreakpointsForDimension1=Controller.R.PC_GS_angles  Table=Controller.R.PC_GS_KI  InternalRulePriority=Speed  RndMeth=Simplest
  1-D Lookup Table2 : Lookup_n-D  NumberOfTableDimensions=1  BreakpointsForDimension1=Controller.R.PC_GS_angles  Table=Controller.R.PC_GS_KP  InternalRulePriority=Speed  RndMeth=Simplest
  Add : Sum
  Add1 : Sum
  Constant1 : Constant  Value=90*pi/180
  Delay : Delay  DelayLength=1  InitialCondition=0
  Gain : Gain  Gain=simu.dt
  Product : Product
  Product1 : Product
  Saturation Dynamic : simulink/Discontinuities/Saturation Dynamic  OutMin=[]  OutMax=[]  OutDataTypeStr=Inherit: Same as second input  OutDataType=fixdt(1, 16)  OutScaling=2^-10  DoSatur=off
  Saturation1 : Saturate  UpperLimit=Controller.R.PC_GS_KI(end)  LowerLimit=Controller.R.PC_GS_KI(1)
  Saturation3 : Saturate  UpperLimit=Controller.R.PC_GS_KP(end)  LowerLimit=Controller.R.PC_GS_KP(1)
  Out1 : Outport
  wires:
  Product/1 -> Add1/1
  Add1/1 -> Out1/1
  Delay/1 -> Add/2
  Saturation Dynamic/1 -> Delay/1, Add1/2
  Constant1/1 -> Saturation Dynamic/1
  In3/1 -> Saturation Dynamic/3
  Add/1 -> Saturation Dynamic/2
  Gain/1 -> Add/1
  Product1/1 -> Gain/1
  Saturation1/1 -> Product1/2
  Saturation3/1 -> Product/2
  In1/1 -> Product1/1, Product/1
  In2/1 -> 1-D Lookup Table2/1, 1-D Lookup Table1/1
  1-D Lookup Table2/1 -> Saturation3/1
  1-D Lookup Table1/1 -> Saturation1/1
